simulink model "Modelo_con_no_linealidades_foto"  (R2020a)
settings: Solver=ode15s  StartTime=0.0  StopTime=10  FixedStep=0.001  MaxStep=0.001  RelTol=1e-3
undefined symbols (not defined in the file): A, Amp, B, ba, Cc, D, f0, fs, g, I_max, K_motor_virtual, ksi, ksia, L, R, R_control, v0, w_acc, x0, zita_acc, ZOH
libraries: simulink x1, dspstat3 x1
settings Model: Creator=Noxi-PC  LastModifiedBy=Noxi-PC

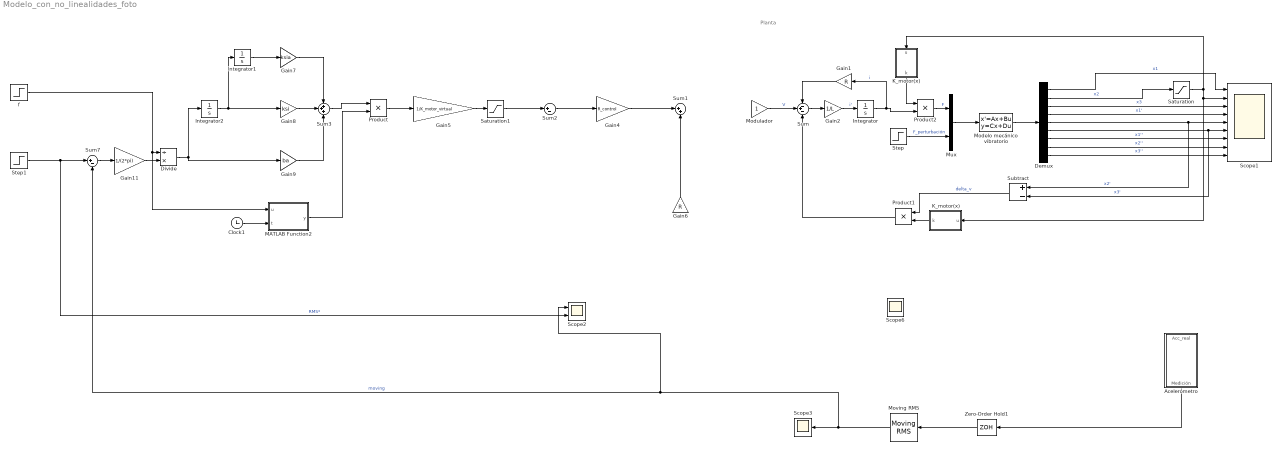
== system Modelo_con_no_linealidades_foto ==
  note: Planta
  " K_motor(x)" : MATLAB Function  TreatAsAtomicUnit=on
  Acelerómetro : Subsystem
  Clock1 : Clock
  Demux : Demux  Outputs=9
  Divide : Product  Inputs=/*
  Gain1 : Gain  Gain=R
  Gain11 : Gain  Gain=1/(2*pi)
  Gain2 : Gain  Gain=1/L
  Gain4 : Gain  Gain=R_control
  Gain5 : Gain  Gain=1/K_motor_virtual
  Gain6 : Gain  Gain=R
  Gain7 : Gain  Gain=ksia
  Gain8 : Gain  Gain=ksi
  Gain9 : Gain  Gain=ba
  Integrator : Integrator
  Integrator1 : Integrator
  Integrator2 : Integrator
  K_motor(x) : MATLAB Function  TreatAsAtomicUnit=on
  MATLAB Function2 : MATLAB Function  TreatAsAtomicUnit=on
  Modelo mecánico vibratorio : StateSpace  A=A  B=B  C=Cc  D=D  InitialCondition=[x0,v0]
  Modulador : Gain
  Moving RMS : dspstat3/Moving RMS  Method=Sliding window  ForgettingFactorPort=off  SpecifyWindowLength=on  WindowLength=Ventana  ForgettingFactor=0.99  SimulateUsing=Code generation
      settings: SourceProductBaseCode=DS
  Mux : Mux  Inputs=2
  Product : Product
  Product1 : Product
  Product2 : Product
  Saturation : Saturate  UpperLimit=12.7e-3  LowerLimit=-12.7e-3
  Saturation1 : Saturate  UpperLimit=I_max  LowerLimit=-I_max
  Scope1 : Scope  NumInputPorts=9
  Scope2 : Scope  NumInputPorts=2
  Scope3 : Scope
  Scope6 : Scope
  Step : Step  Time=3  After=0  SampleTime=0
  Step1 : Step  After=Amp/sqrt(2)  SampleTime=0
  Subtract : Sum  Inputs=+-
  Sum : Sum  Inputs=-+-
  Sum1 : Sum  Inputs=|++
  Sum2 : Sum  Inputs=|+-
  Sum3 : Sum  Inputs=+++
  Sum7 : Sum  Inputs=|+-
  Zero-Order Hold1 : ZeroOrderHold  SampleTime=ZOH
  f : Step  Time=0  After=f0  SampleTime=0
  wires:
  Modelo mecánico vibratorio/1 -> Demux/1
  Demux/1 -> Scope1/1  "x1"
  Demux/2 -> Saturation/1  "x2"
  Demux/3 -> Scope1/3  "x3"
  Demux/4 -> Scope1/4  "x1'"
  Demux/5 -> Scope1/5, Subtract/1  "x2'"
  Demux/6 -> Scope1/6, Subtract/2  "x3'"
  Demux/7 -> Scope1/7  "x1''"
  Demux/8 -> Scope1/8  "x2''"
  Demux/9 -> Scope1/9  "x3''"
  Mux/1 -> Modelo mecánico vibratorio/1
  Sum/1 -> Gain2/1
  Integrator/1 -> Product2/2, Gain1/1  "i"
  Gain1/1 -> Sum/1
  Gain2/1 -> Integrator/1  "i'"
  Step/1 -> Mux/2  "F_perturbación"
  Product1/1 -> Sum/3
  Subtract/1 -> Product1/1  "delta_v"
  Modulador/1 -> Sum/2  "V"
  Sum2/1 -> Gain4/1
  Gain5/1 -> Saturation1/1
  Gain4/1 -> Sum1/1
  Gain8/1 -> Sum3/2
  Gain7/1 -> Sum3/1
  Gain9/1 -> Sum3/3
  Integrator1/1 -> Gain7/1
  Integrator2/1 -> Integrator1/1, Gain8/1
  Acelerómetro/1(Medición) -> Zero-Order Hold1/1
  Zero-Order Hold1/1 -> Moving RMS/1
  Step1/1 -> Scope2/2, Sum7/1  "RMS*"
  Moving RMS/1 -> Scope2/1, Sum7/2, Scope3/1  "moving"
  Sum7/1 -> Gain11/1
  Sum3/1 -> Product/1
  Saturation/1 -> " K_motor(x)"/1(u), Scope1/2, K_motor(x)/1(u)
  Product2/1 -> Mux/1  "F"
  K_motor(x)/1(k) -> Product2/1
  " K_motor(x)"/1(k) -> Product1/2
  Divide/1 -> Gain9/1, Integrator2/1
  Gain11/1 -> Divide/2
  Product/1 -> Gain5/1
  Saturation1/1 -> Sum2/1
  f/1 -> MATLAB Function2/1(u), Divide/1
  MATLAB Function2/1(y) -> Product/2
  Clock1/1 -> MATLAB Function2/2(t)
  Gain6/1 -> Sum1/2

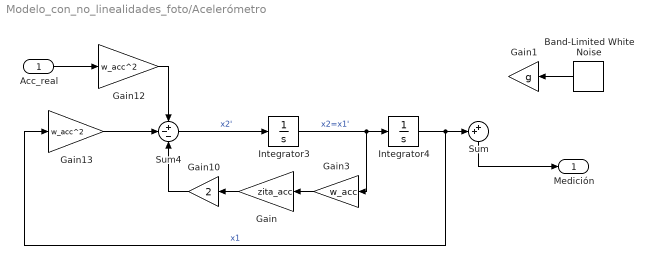
== system Modelo_con_no_linealidades_foto/Acelerómetro ==
  Acc_real : Inport
  Band-Limited White Noise : simulink/Sources/Band-Limited White Noise  Cov=NoisePower  Ts=1/fs  seed=[23341]
  Gain : Gain  Gain=zita_acc
  Gain1 : Gain  Gain=g
  Gain10 : Gain  Gain=2
  Gain12 : Gain  Gain=w_acc^2
  Gain13 : Gain  Gain=w_acc^2
  Gain3 : Gain  Gain=w_acc
  Integrator3 : Integrator
  Integrator4 : Integrator
  Sum : Sum  Inputs=++|
  Sum4 : Sum  Inputs=+--
  Medición : Outport
  wires:
  Gain/1 -> Gain10/1
  Integrator4/1 -> Gain13/1, Sum/1  "x1"
  Acc_real/1 -> Gain12/1
  Gain12/1 -> Sum4/1
  Sum4/1 -> Integrator3/1  "x2'"
  Gain3/1 -> Gain/1
  Integrator3/1 -> Integrator4/1, Gain3/1  "x2=x1'"
  Gain13/1 -> Sum4/2
  Gain10/1 -> Sum4/3
  Band-Limited White Noise/1 -> Gain1/1
  Sum/1 -> Medición/1

== matlab function Modelo_con_no_linealidades_foto/ K_motor(x) ==
  data: u input; k output
function k= fcn(u)
coefs = [1883883250149.81,121220914.941173,-604988778.285297,-369001.905871325,-43371.4523559472,-47.4444922489166,51.4222931299995];

k = coefs(1)*u^6+coefs(2)*u^5+coefs(3)*u^4+coefs(4)*u^3+coefs(5)*u^2+coefs(6)*u^1+coefs(7);

== matlab function Modelo_con_no_linealidades_foto/MATLAB Function2 ==
  data: u input; y output; t input
function y = fcn(u,t)

y = sin(2*pi*u*t);

== matlab function Modelo_con_no_linealidades_foto/K_motor(x) ==
  data: u input; k output
function k = fcn(u)
coefs = [1.88388325014986e-06,1.21220914940963e-07,-0.000604988778285308,-0.000369001905871298,-0.0433714523559467,-0.0474444922489168,51.4222931299995];

k = coefs(1)*u^6+coefs(2)*u^5+coefs(3)*u^4+coefs(4)*u^3+coefs(5)*u^2+coefs(6)*u^1+coefs(7);
